simulink model "Observer_Harness"  (R2023a)
settings: Solver=ode23t  StartTime=0.0  StopTime=1  MaxStep=0.1  RelTol=1e-4
libraries: SignalEditorBlockLib x1
settings Model: Creator=ПК  LastModifiedBy=ПК

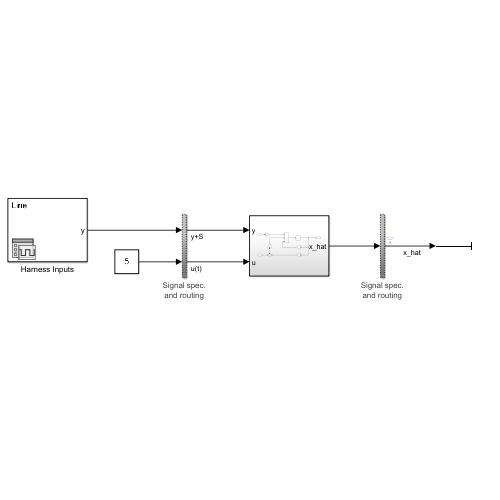
[thumbnail: Simulink's stored preview of the top-level diagram]
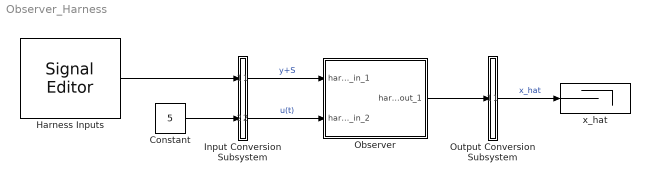
== system Observer_Harness ==
  Constant : Constant  Value=5
  Harness Inputs : SignalEditorBlockLib/Signal Editor  FileName=C:\Users\ПК\Desktop\Work\BMSTU\6 сем\ТАУ\Theory-of-Automatic-Control\Lab-7\tests\Observer_Harness_HarnessInputs.mat  ActiveScenario=Line  ActiveSignal=y  IsBus=off  OutputBusObjectStr=Bus: BusObject  SampleTime=0  Interpolate=off  ZeroCross=off  OutputAfterFinalValue=Setting to zero  Unit=inherit  PreserveSignalName=on  ApplySigPropsToAllScenarios=on
  Input Conversion Subsystem : Subsystem  Tag=__SLT_ICS__  Description=|
      | Signal spec.
      | and routing
      settings: AttributesFormatString=%<Description>
  Observer : Subsystem  Tag=__SL_testing_harness_stub_
  Output Conversion Subsystem : Subsystem  Tag=__SLT_OCS__  Description=|
      | Signal spec.
      | and routing
      settings: AttributesFormatString=%<Description>
  x_hat : Terminator
  wires:
  Harness Inputs/1 -> Input Conversion Subsystem/1(Inport_1)
  Constant/1 -> Input Conversion Subsystem/2(Inport_2)
  Output Conversion Subsystem/1(Outport_1) -> x_hat/1  "x_hat"
  Input Conversion Subsystem/1(Outport_1) -> Observer/1(harness_in_1)  "y+S"
  Input Conversion Subsystem/2(Outport_2) -> Observer/2(harness_in_2)  "u(t)"
  Observer/1(harness_out_1) -> Output Conversion Subsystem/1(Inport_1)

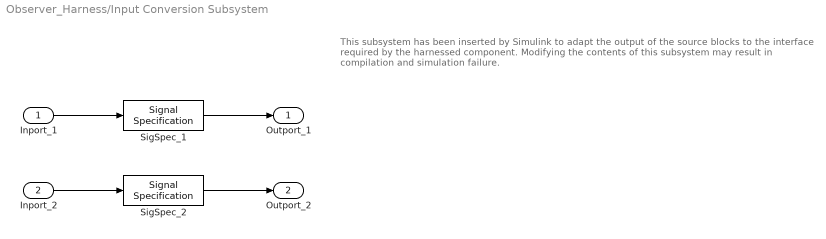
== system Observer_Harness/Input Conversion Subsystem ==
  note: This subsystem has been inserted by Simulink to adapt the output of the source blocks to the interface required by the harnessed component.
      |  Modifying the contents of this subsystem may result in compilation and simulation failure.
  Inport_1 : Inport
  Inport_2 : Inport  Port=2
  SigSpec_1 : SignalSpecification  OutDataTypeStr=double  Dimensions=[1]  SampleTime=[0, 0]
  SigSpec_2 : SignalSpecification  OutDataTypeStr=double  Dimensions=[1]  SampleTime=[0, 0]
  Outport_1 : Outport
  Outport_2 : Outport  Port=2
  wires:
  SigSpec_1/1 -> Outport_1/1
  Inport_1/1 -> SigSpec_1/1
  SigSpec_2/1 -> Outport_2/1
  Inport_2/1 -> SigSpec_2/1

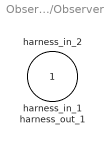
== system Observer_Harness/Observer ==
  harness_in_1 : Inport
  harness_in_2 : Inport  Port=2
  harness_out_1 : Outport

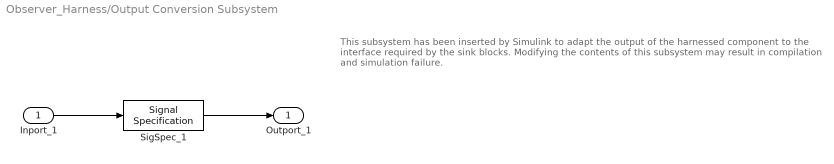
== system Observer_Harness/Output Conversion Subsystem ==
  note: This subsystem has been inserted by Simulink to adapt the output of the harnessed component to the interface required by the sink blocks.
      |  Modifying the contents of this subsystem may result in compilation and simulation failure.
  Inport_1 : Inport
  SigSpec_1 : SignalSpecification  OutDataTypeStr=double  Dimensions=[3]
  Outport_1 : Outport
  wires:
  Inport_1/1 -> SigSpec_1/1
  SigSpec_1/1 -> Outport_1/1
